simulink subsystem "Polynomial_Fitting"  (R2022b)
settings: Solver=VariableStepAuto  StartTime=0.0  StopTime=10.0  RelTol=1e-3
settings Model: Creator=User  LastModifiedBy=User

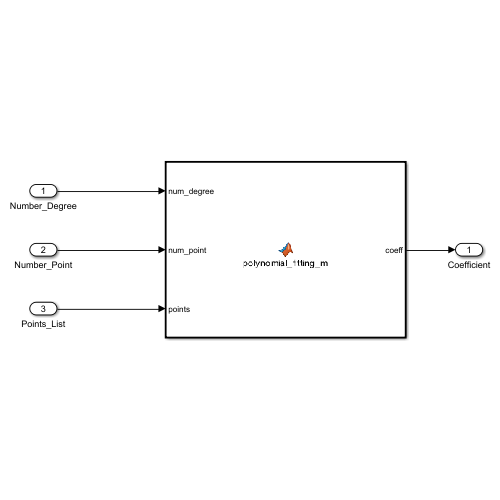
[thumbnail: Simulink's stored preview of the top-level diagram]
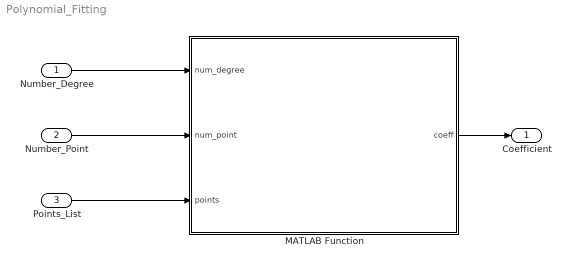
== system Polynomial_Fitting ==
  Number_Degree : Inport
  Number_Point : Inport  Port=2
  Points_List : Inport  Port=3
  MATLAB Function : MATLAB Function  TreatAsAtomicUnit=on
  Coefficient : Outport
  wires:
  Number_Degree/1 -> MATLAB Function/1(num_degree)
  Number_Point/1 -> MATLAB Function/2(num_point)
  Points_List/1 -> MATLAB Function/3(points)
  MATLAB Function/1(coeff) -> Coefficient/1

== matlab function Polynomial_Fitting/MATLAB Function ==
  data: num_degree input; coeff output; num_point input; points input
function coeff = polynomial_fitting_m(num_degree, num_point, points)
    coeff = polynomial_fitting(num_degree, num_point, points);
    
end
